simulink model "nn_fuel_control_4_15"  (R2021a)
settings: Solver=ode15s  StartTime=0.0  StopTime=T  MaxStep=.01  RelTol=1e-3
undefined symbols (not defined in the file): AF_sensor_tol, fault_time, fuel_inj_tol, kappa_tol, MAF_sensor_tol, pump_tol, tau_ww_tol
libraries: neural x66
(part 2 of 3)

== system nn_fuel_control_4_15/Air Fuel Control Model 1/Feed-Forward Neural Network/Layer 2/Delays 1 ==
  "p{2}" : Inport  PortDimensions=15
      mask Display: e = 0.06;c1 = [120 230 180]/255;c2 = ([120 230 180]+0)/(256+128);c3 = ([120 230 180]+128)/(256+128);patch([0 1 1 0],[0 0 1 1],c1);patch([0 1 1 1-e 1-e 0+e],[0 0 1 1-e 0+e 0+e],c2);patch([0 0 1 1-e 0+e 0+e],[0 1 1 1-e 1-e 0+e],c3);plot([0 1 1 0 0],[0 0 1 1 0]);
  mux : Mux  Inputs=1
      mask Display: e = 0.06;c1 = [120 150 230]/255;c2 = ([120 150 230]+0)/383;c3 = ([120 150 230]+128)/383;patch([0 1 1 0],[0 0 1 1],c1);patch([0 1 1 1-e 1-e 0+e],[0 0 1 1-e 0+e 0+e],c2);patch([0 0 1 1-e 0+e 0+e],[0 1 1 1-e 1-e 0+e],c3);plot([0 1 1 0 0],[0 0 1 1 0]);disp('Mux')
  "pd{2,1}" : Outport
      mask Display: e = 0.06;c1 = [120 230 180]/255;c2 = ([120 230 180]+0)/(256+128);c3 = ([120 230 180]+128)/(256+128);patch([0 1 1 0],[0 0 1 1],c1);patch([0 1 1 1-e 1-e 0+e],[0 0 1 1-e 0+e 0+e],c2);patch([0 0 1 1-e 0+e 0+e],[0 1 1 1-e 1-e 0+e],c3);plot([0 1 1 0 0],[0 0 1 1 0]);
  wires:
  "p{2}"/1 -> mux/1
  mux/1 -> "pd{2,1}"/1

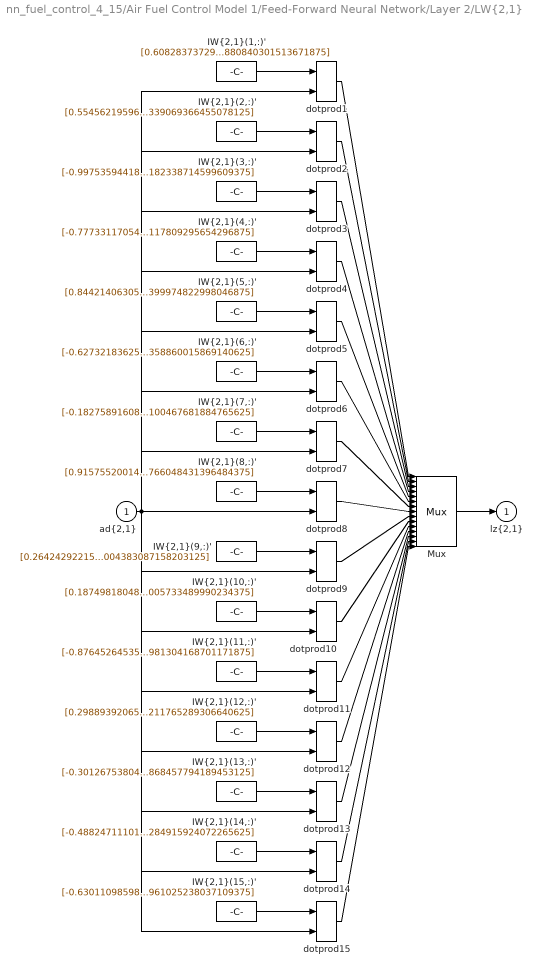
== system nn_fuel_control_4_15/Air Fuel Control Model 1/Feed-Forward Neural Network/Layer 2/LW{2,1} ==
  "ad{2,1}" : Inport  PortDimensions=15
      mask Display: e = 0.06;c1 = [120 230 180]/255;c2 = ([120 230 180]+0)/(256+128);c3 = ([120 230 180]+128)/(256+128);patch([0 1 1 0],[0 0 1 1],c1);patch([0 1 1 1-e 1-e 0+e],[0 0 1 1-e 0+e 0+e],c2);patch([0 0 1 1-e 0+e 0+e],[0 1 1 1-e 1-e 0+e],c3);plot([0 1 1 0 0],[0 0 1 1 0]);
  "IW{2,1}(1,:)'" : Constant  Value=[0.60828373729495710531267604892491362988948822021484375;0.1631652431061806074463760296566761098802089691162109375;-0.44374590709596450910368048425880260765552520751953125;0.345526680299295285703209401617641560733318328857421875;0.348097898689621876311406367676681838929653167724609375;0.8265636312091990678396768998936749994754791259765625;-0.01586618016159375976759093873624806292355060577392578125;0.6795632649425040749946447249385528266429901123046875;0.75459019889386735879810430560610257089138031005859375;-0.94837435293727867513524643072742037475109100341796875;-0.14339378395662694121170943617471493780612945556640625;0.1155478101778000254995504292310215532779693603515625;0.032676095155037145068011028570253984071314334869384765625;0.719801219521268631496013767900876700878143310546875;-0.5649534439609567026963077296386472880840301513671875]
      mask Display: e = 0.06;c1 = [120 150 230]/255;c2 = ([120 150 230]+0)/383;c3 = ([120 150 230]+128)/383;patch([0 1 1 0],[0 0 1 1],c1);patch([0 1 1 1-e 1-e 0+e],[0 0 1 1-e 0+e 0+e],c2);patch([0 0 1 1-e 0+e 0+e],[0 1 1 1-e 1-e 0+e],c3);plot([0 1 1 0 0],[0 0 1 1 0]);disp('weights');
  "IW{2,1}(10,:)'" : Constant  Value=[0.1874981804874335244992522575557813979685306549072265625;-0.387364613522674650081256686462438665330410003662109375;0.78290743200496437648183700730442069470882415771484375;0.86317824192602399246965205747983418405055999755859375;-0.59813734503873805525842044517048634588718414306640625;0.3906864891603387679452907832455821335315704345703125;-0.8173791825222698204100879593170247972011566162109375;0.9015721689759768064931222397717647254467010498046875;-0.146378292631031692305754177141352556645870208740234375;0.53947856391638715489733613139833323657512664794921875;-0.709668238586643074228277328074909746646881103515625;0.04455141979717640310365567302142153494060039520263671875;0.6061687426195963013242362649179995059967041015625;0.0751321602491212825469801828148774802684783935546875;0.478851095922558922524103763862513005733489990234375]
      mask Display: e = 0.06;c1 = [120 150 230]/255;c2 = ([120 150 230]+0)/383;c3 = ([120 150 230]+128)/383;patch([0 1 1 0],[0 0 1 1],c1);patch([0 1 1 1-e 1-e 0+e],[0 0 1 1-e 0+e 0+e],c2);patch([0 0 1 1-e 0+e 0+e],[0 1 1 1-e 1-e 0+e],c3);plot([0 1 1 0 0],[0 0 1 1 0]);disp('weights');
  "IW{2,1}(11,:)'" : Constant  Value=[-0.87645264535886735490777255108696408569812774658203125;-0.354803487782416215878811271977610886096954345703125;0.89745590027941080091267167517798952758312225341796875;0.12153107756977178655066751389313139952719211578369140625;0.0263130815585567445769044070402742363512516021728515625;-0.809370187848432731669845452415756881237030029296875;-0.50487186526927352314686459067161194980144500732421875;0.263576711957190124024918986833654344081878662109375;0.7429357474631868019088187793386168777942657470703125;0.12413592320170453719985204088516184128820896148681640625;0.12395570443307211971895043234326294623315334320068359375;-0.09320289501976443402586625097683281637728214263916015625;0.2053486431587812355292754773472552187740802764892578125;-0.14973778798840076120768571854569017887115478515625;-0.935185280441018118580132068018428981304168701171875]
      mask Display: e = 0.06;c1 = [120 150 230]/255;c2 = ([120 150 230]+0)/383;c3 = ([120 150 230]+128)/383;patch([0 1 1 0],[0 0 1 1],c1);patch([0 1 1 1-e 1-e 0+e],[0 0 1 1-e 0+e 0+e],c2);patch([0 0 1 1-e 0+e 0+e],[0 1 1 1-e 1-e 0+e],c3);plot([0 1 1 0 0],[0 0 1 1 0]);disp('weights');
  "IW{2,1}(12,:)'" : Constant  Value=[0.298893920656925160539429953132639639079570770263671875;-0.943158196479241706100538067403249442577362060546875;-0.72901934273769131156228695544996298849582672119140625;-0.4420743609879778102111913540284149348735809326171875;0.162898079805751105908484532847069203853607177734375;-0.03893962992941624179366044700145721435546875;-0.0249149427296144754251372432918287813663482666015625;0.7848685910094259643443592722178436815738677978515625;-0.7452172890261443694015497385407797992229461669921875;0.5937912927176427491104959699441678822040557861328125;-0.6901888632454264982385438997880555689334869384765625;0.297856720876973513068008969639777205884456634521484375;0.5644902002231066973081397009082138538360595703125;-0.1919252452819204535217068041674792766571044921875;0.955896418076493947779681548126973211765289306640625]
      mask Display: e = 0.06;c1 = [120 150 230]/255;c2 = ([120 150 230]+0)/383;c3 = ([120 150 230]+128)/383;patch([0 1 1 0],[0 0 1 1],c1);patch([0 1 1 1-e 1-e 0+e],[0 0 1 1-e 0+e 0+e],c2);patch([0 0 1 1-e 0+e 0+e],[0 1 1 1-e 1-e 0+e],c3);plot([0 1 1 0 0],[0 0 1 1 0]);disp('weights');
  "IW{2,1}(13,:)'" : Constant  Value=[-0.301267538043442584250186655481229536235332489013671875;0.2137960673758446950021294696853146888315677642822265625;-0.6099118162917822605351148013141937553882598876953125;-0.804913922659836078565831485320813953876495361328125;-0.77569083568485186486185511967050842940807342529296875;-0.1203229492733475236576623501605354249477386474609375;-0.4309096198696529267380128658260218799114227294921875;0.4020616862706465344245998494443483650684356689453125;0.8648307403643740176590881674201227724552154541015625;-0.7468845527558245489530008853762410581111907958984375;0.856263604397531796763587408349849283695220947265625;-0.9225328397592240659008666625595651566982269287109375;0.9259027011481022473304847153485752642154693603515625;0.567169309423982692663912530406378209590911865234375;-0.2729640593072322207746083222446031868457794189453125]
      mask Display: e = 0.06;c1 = [120 150 230]/255;c2 = ([120 150 230]+0)/383;c3 = ([120 150 230]+128)/383;patch([0 1 1 0],[0 0 1 1],c1);patch([0 1 1 1-e 1-e 0+e],[0 0 1 1-e 0+e 0+e],c2);patch([0 0 1 1-e 0+e 0+e],[0 1 1 1-e 1-e 0+e],c3);plot([0 1 1 0 0],[0 0 1 1 0]);disp('weights');
  "IW{2,1}(14,:)'" : Constant  Value=[-0.4882471110167276862057406106032431125640869140625;-0.153288731021647084418191298027522861957550048828125;0.42935429919651912911149338469840586185455322265625;-0.9702630312509814558552534435875713825225830078125;0.3583641699961483961800468023284338414669036865234375;-0.1353416572083896429745664136135019361972808837890625;0.4918952919432595383142370337736792862415313720703125;-0.57640236234023856098929172731004655361175537109375;-0.8508523606948406037275844937539659440517425537109375;-0.0224638760367827927666439791209995746612548828125;-0.095033702909726347485275255166925489902496337890625;0.8424006088431996719378958005108870565891265869140625;-0.6849380364954396060994668005150742828845977783203125;0.6228510334032935080728066168376244604587554931640625;-0.4631992710325454343234241605387069284915924072265625]
      mask Display: e = 0.06;c1 = [120 150 230]/255;c2 = ([120 150 230]+0)/383;c3 = ([120 150 230]+128)/383;patch([0 1 1 0],[0 0 1 1],c1);patch([0 1 1 1-e 1-e 0+e],[0 0 1 1-e 0+e 0+e],c2);patch([0 0 1 1-e 0+e 0+e],[0 1 1 1-e 1-e 0+e],c3);plot([0 1 1 0 0],[0 0 1 1 0]);disp('weights');
  "IW{2,1}(15,:)'" : Constant  Value=[-0.630110985981365612218496607965789735317230224609375;0.8242276349657886580502008655457757413387298583984375;-0.400759189777235125262677684077061712741851806640625;0.3277466841598546398728331041638739407062530517578125;0.8915540017782561665882212764699943363666534423828125;0.83874918710984758263293770141899585723876953125;0.45485624724982631761349693988449871540069580078125;0.4460472529162602395302883451222442090511322021484375;0.093826789799659859880875956150703132152557373046875;-0.9259823634579957829515706180245615541934967041015625;0.402471624402540584242160548456013202667236328125;-0.3445278733840286822243115238961763679981231689453125;-0.74855326961618029457667944370768964290618896484375;0.95153598362676117261571562266908586025238037109375;0.9375332121621331449290437376475892961025238037109375]
      mask Display: e = 0.06;c1 = [120 150 230]/255;c2 = ([120 150 230]+0)/383;c3 = ([120 150 230]+128)/383;patch([0 1 1 0],[0 0 1 1],c1);patch([0 1 1 1-e 1-e 0+e],[0 0 1 1-e 0+e 0+e],c2);patch([0 0 1 1-e 0+e 0+e],[0 1 1 1-e 1-e 0+e],c3);plot([0 1 1 0 0],[0 0 1 1 0]);disp('weights');
  "IW{2,1}(2,:)'" : Constant  Value=[0.554562195967324811363141634501516819000244140625;0.1497692577584186779393604638244141824543476104736328125;0.56295505738794149319659254615544341504573822021484375;-0.79339302952488333087188721037819050252437591552734375;-0.5227228745047407532098304727696813642978668212890625;-0.3416227507267695084891556689399294555187225341796875;-0.077931032288060197998902367544360458850860595703125;0.791132526371828515010520277428440749645233154296875;-0.58148454694741247283928942124475724995136260986328125;0.141240162213906061960955184986232779920101165771484375;-0.47295622510494939039205064545967616140842437744140625;-0.88474738325846635778049176224158145487308502197265625;-0.2412424077947986911230060513844364322721958160400390625;0.026695649520263042830947597394697368144989013671875;-0.168815586171824794092799493228085339069366455078125]
      mask Display: e = 0.06;c1 = [120 150 230]/255;c2 = ([120 150 230]+0)/383;c3 = ([120 150 230]+128)/383;patch([0 1 1 0],[0 0 1 1],c1);patch([0 1 1 1-e 1-e 0+e],[0 0 1 1-e 0+e 0+e],c2);patch([0 0 1 1-e 0+e 0+e],[0 1 1 1-e 1-e 0+e],c3);plot([0 1 1 0 0],[0 0 1 1 0]);disp('weights');
  "IW{2,1}(3,:)'" : Constant  Value=[-0.997535944186512590903248565155081450939178466796875;0.9844775557991563008641833221190609037876129150390625;0.13365057898997889651582227088510990142822265625;0.598462918022267142958980912226252257823944091796875;-0.6928984585121236161597835234715603291988372802734375;0.47725275298145408697791935992427170276641845703125;0.31490478145201183934887012583203613758087158203125;-0.596507724440733522186519621754996478557586669921875;0.00503819451104714488565150531940162181854248046875;-0.1558413435872125774039886891841888427734375;0.069703488503479515969729618518613278865814208984375;0.252706700102361292437080919626168906688690185546875;0.6096076508018011264056212894502095878124237060546875;-0.6419028490453777546775882001384161412715911865234375;0.809099317995565225913878748542629182338714599609375]
      mask Display: e = 0.06;c1 = [120 150 230]/255;c2 = ([120 150 230]+0)/383;c3 = ([120 150 230]+128)/383;patch([0 1 1 0],[0 0 1 1],c1);patch([0 1 1 1-e 1-e 0+e],[0 0 1 1-e 0+e 0+e],c2);patch([0 0 1 1-e 0+e 0+e],[0 1 1 1-e 1-e 0+e],c3);plot([0 1 1 0 0],[0 0 1 1 0]);disp('weights');
  "IW{2,1}(4,:)'" : Constant  Value=[-0.7773311705499761359305921359919011592864990234375;-0.1463969306597807662484456159290857613086700439453125;-0.52098250625950992542811945895664393901824951171875;0.1340370775561925409391506036627106368541717529296875;0.286894704491670982093864950002171099185943603515625;-0.2232587156037413311793216053047217428684234619140625;0.30007640022437698235080461017787456512451171875;-0.587710092220042223942755299503915011882781982421875;0.3578658787775890193216810075682587921619415283203125;-0.2262986592885329883984013576991856098175048828125;-0.658201336972639605704671339481137692928314208984375;-0.2545120319323490587493097336846403777599334716796875;-0.2189509488661911529305825752089731395244598388671875;-0.1927993718650127252800530186505056917667388916015625;0.31411982797593207550335137057118117809295654296875]
      mask Display: e = 0.06;c1 = [120 150 230]/255;c2 = ([120 150 230]+0)/383;c3 = ([120 150 230]+128)/383;patch([0 1 1 0],[0 0 1 1],c1);patch([0 1 1 1-e 1-e 0+e],[0 0 1 1-e 0+e 0+e],c2);patch([0 0 1 1-e 0+e 0+e],[0 1 1 1-e 1-e 0+e],c3);plot([0 1 1 0 0],[0 0 1 1 0]);disp('weights');
  "IW{2,1}(5,:)'" : Constant  Value=[0.8442140630590719840853353161946870386600494384765625;-0.338275289571432880020296352086006663739681243896484375;0.78093285572494230972750983710284344851970672607421875;0.5354024127678302935606780010857619345188140869140625;-0.08976512545403049492254154984038905240595340728759765625;0.0061947204318573145798154655494727194309234619140625;-0.66291433016892231666616908114519901573657989501953125;-0.0206699629090130176933826078311540186405181884765625;-0.59971454427786785590370755016920156776905059814453125;0.10166800703172866604528934431073139421641826629638671875;-0.7738583581044451431552033682237379252910614013671875;0.54327144951764783087355681345798075199127197265625;-0.7895437576381787447843407790060155093669891357421875;-0.264681039126205330802577009308151900768280029296875;-0.531626874309292229980883348616771399974822998046875]
      mask Display: e = 0.06;c1 = [120 150 230]/255;c2 = ([120 150 230]+0)/383;c3 = ([120 150 230]+128)/383;patch([0 1 1 0],[0 0 1 1],c1);patch([0 1 1 1-e 1-e 0+e],[0 0 1 1-e 0+e 0+e],c2);patch([0 0 1 1-e 0+e 0+e],[0 1 1 1-e 1-e 0+e],c3);plot([0 1 1 0 0],[0 0 1 1 0]);disp('weights');
  "IW{2,1}(6,:)'" : Constant  Value=[-0.6273218362596340025305607923655770719051361083984375;0.656185430676088810031387765775434672832489013671875;0.811438500319960898110593916499055922031402587890625;0.6995755518931172645125116105191409587860107421875;-0.1562054093044125957501222501377924345433712005615234375;-0.0322626762571427416759206607821397483348846435546875;-0.01132390864387658978296169465238563134334981441497802734375;-0.4057941893418341994248521586996503174304962158203125;0.70209822919968012389091427394305355846881866455078125;-0.6537984598108443901054442903841845691204071044921875;-0.53447697884651301780678522845846600830554962158203125;0.9945723398383783386833556505735032260417938232421875;-0.168349065817595733296485605023917742073535919189453125;-0.164941923712752736008724241401068866252899169921875;0.071348316420243751423413414158858358860015869140625]
      mask Display: e = 0.06;c1 = [120 150 230]/255;c2 = ([120 150 230]+0)/383;c3 = ([120 150 230]+128)/383;patch([0 1 1 0],[0 0 1 1],c1);patch([0 1 1 1-e 1-e 0+e],[0 0 1 1-e 0+e 0+e],c2);patch([0 0 1 1-e 0+e 0+e],[0 1 1 1-e 1-e 0+e],c3);plot([0 1 1 0 0],[0 0 1 1 0]);disp('weights');
  "IW{2,1}(7,:)'" : Constant  Value=[-0.1827589160867006956578961762716062366962432861328125;0.264553209549575729653270173002965748310089111328125;-0.602076083278996865288945627980865538120269775390625;-0.8668388126716621844281007724930532276630401611328125;-0.631703471288605822309136783587746322154998779296875;0.738811602164048064622647871146909892559051513671875;-0.29851980211238693385666920221410691738128662109375;-0.9066514471495474847273499108268879354000091552734375;0.7667373784025228733440826545120216906070709228515625;-0.8003713287638996032313798423274420201778411865234375;0.572112014899465837203251794562675058841705322265625;0.0556726723526870248548448216752149164676666259765625;0.1886458668441315378316858186735771596431732177734375;-0.43769519159423087018012665794230997562408447265625;0.2958829770965698546802968849078752100467681884765625]
      mask Display: e = 0.06;c1 = [120 150 230]/255;c2 = ([120 150 230]+0)/383;c3 = ([120 150 230]+128)/383;patch([0 1 1 0],[0 0 1 1],c1);patch([0 1 1 1-e 1-e 0+e],[0 0 1 1-e 0+e 0+e],c2);patch([0 0 1 1-e 0+e 0+e],[0 1 1 1-e 1-e 0+e],c3);plot([0 1 1 0 0],[0 0 1 1 0]);disp('weights');
  "IW{2,1}(8,:)'" : Constant  Value=[0.9157552001415154574459620562265627086162567138671875;0.1691210332467132648748275869365897960960865020751953125;-0.410972009283113226540962159560876898467540740966796875;-0.79231054870772366083286897264770232141017913818359375;-0.6664760715628090803619443249772302806377410888671875;0.4958051958545179882520415048929862678050994873046875;0.8372202716459440363649946448276750743389129638671875;-0.6574527075494429606550284006516449153423309326171875;0.20364663569650731655968911582021974027156829833984375;0.477164411668982768599533983433502726256847381591796875;0.2366940977861309580720927669972297735512256622314453125;-0.137137595850200855185363479904481209814548492431640625;-0.0219191390002913925882932488775622914545238018035888671875;-0.414790307653978285173934636986814439296722412109375;0.2688907245261178413642255691229365766048431396484375]
      mask Display: e = 0.06;c1 = [120 150 230]/255;c2 = ([120 150 230]+0)/383;c3 = ([120 150 230]+128)/383;patch([0 1 1 0],[0 0 1 1],c1);patch([0 1 1 1-e 1-e 0+e],[0 0 1 1-e 0+e 0+e],c2);patch([0 0 1 1-e 0+e 0+e],[0 1 1 1-e 1-e 0+e],c3);plot([0 1 1 0 0],[0 0 1 1 0]);disp('weights');
  "IW{2,1}(9,:)'" : Constant  Value=[0.264242922159276749649592375135398469865322113037109375;0.0281964884631230143507973906480401637963950634002685546875;0.437970352052139799692298538502654992043972015380859375;0.85719086127498778093780629205866716802120208740234375;0.6149400332096350840771492585190571844577789306640625;-0.1298886743902054607957552434527315199375152587890625;-0.116547252626436392830555632826872169971466064453125;-0.99659741931905632128518846002407371997833251953125;-0.19318002865432382098020980265573598444461822509765625;-0.8425582572983163487378988065756857395172119140625;0.1149262515205252410677161378771415911614894866943359375;0.73176535852285640171288605415611527860164642333984375;-0.2544570268941874768842126286472193896770477294921875;0.66147788735934387460702055250294506549835205078125;-0.688203072177270502862711509806104004383087158203125]
      mask Display: e = 0.06;c1 = [120 150 230]/255;c2 = ([120 150 230]+0)/383;c3 = ([120 150 230]+128)/383;patch([0 1 1 0],[0 0 1 1],c1);patch([0 1 1 1-e 1-e 0+e],[0 0 1 1-e 0+e 0+e],c2);patch([0 0 1 1-e 0+e 0+e],[0 1 1 1-e 1-e 0+e],c3);plot([0 1 1 0 0],[0 0 1 1 0]);disp('weights');
  Mux : Mux  Inputs=15
      mask Display: e = 0.06;c1 = [120 150 230]/255;c2 = ([120 150 230]+0)/383;c3 = ([120 150 230]+128)/383;patch([0 1 1 0],[0 0 1 1],c1);patch([0 1 1 1-e 1-e 0+e],[0 0 1 1-e 0+e 0+e],c2);patch([0 0 1 1-e 0+e 0+e],[0 1 1 1-e 1-e 0+e],c3);plot([0 1 1 0 0],[0 0 1 1 0]);disp('Mux');
  dotprod{1..15} (15 alike) : neural/Weight Functions/dotprod
  "lz{2,1}" : Outport
      mask Display: e = 0.06;c1 = [120 230 180]/255;c2 = ([120 230 180]+0)/(256+128);c3 = ([120 230 180]+128)/(256+128);patch([0 1 1 0],[0 0 1 1],c1);patch([0 1 1 1-e 1-e 0+e],[0 0 1 1-e 0+e 0+e],c2);patch([0 0 1 1-e 0+e 0+e],[0 1 1 1-e 1-e 0+e],c3);plot([0 1 1 0 0],[0 0 1 1 0]);
  wires:
  "IW{2,1}(1,:)'"/1 -> dotprod1/1
  "ad{2,1}"/1 -> dotprod1/2, dotprod2/2, dotprod3/2, dotprod4/2, dotprod5/2, dotprod6/2, dotprod7/2, dotprod8/2, dotprod9/2, dotprod10/2, dotprod11/2, dotprod12/2, dotprod13/2, dotprod14/2, dotprod15/2
  dotprod1/1 -> Mux/1
  "IW{2,1}(2,:)'"/1 -> dotprod2/1
  dotprod2/1 -> Mux/2
  "IW{2,1}(3,:)'"/1 -> dotprod3/1
  dotprod3/1 -> Mux/3
  "IW{2,1}(4,:)'"/1 -> dotprod4/1
  dotprod4/1 -> Mux/4
  "IW{2,1}(5,:)'"/1 -> dotprod5/1
  dotprod5/1 -> Mux/5
  "IW{2,1}(6,:)'"/1 -> dotprod6/1
  dotprod6/1 -> Mux/6
  "IW{2,1}(7,:)'"/1 -> dotprod7/1
  dotprod7/1 -> Mux/7
  "IW{2,1}(8,:)'"/1 -> dotprod8/1
  dotprod8/1 -> Mux/8
  "IW{2,1}(9,:)'"/1 -> dotprod9/1
  dotprod9/1 -> Mux/9
  "IW{2,1}(10,:)'"/1 -> dotprod10/1
  dotprod10/1 -> Mux/10
  "IW{2,1}(11,:)'"/1 -> dotprod11/1
  dotprod11/1 -> Mux/11
  "IW{2,1}(12,:)'"/1 -> dotprod12/1
  dotprod12/1 -> Mux/12
  "IW{2,1}(13,:)'"/1 -> dotprod13/1
  dotprod13/1 -> Mux/13
  "IW{2,1}(14,:)'"/1 -> dotprod14/1
  dotprod14/1 -> Mux/14
  "IW{2,1}(15,:)'"/1 -> dotprod15/1
  dotprod15/1 -> Mux/15
  Mux/1 -> "lz{2,1}"/1

== system nn_fuel_control_4_15/Air Fuel Control Model 1/Feed-Forward Neural Network/Layer 3/Delays 1 ==
  "p{3}" : Inport  PortDimensions=15
      mask Display: e = 0.06;c1 = [120 230 180]/255;c2 = ([120 230 180]+0)/(256+128);c3 = ([120 230 180]+128)/(256+128);patch([0 1 1 0],[0 0 1 1],c1);patch([0 1 1 1-e 1-e 0+e],[0 0 1 1-e 0+e 0+e],c2);patch([0 0 1 1-e 0+e 0+e],[0 1 1 1-e 1-e 0+e],c3);plot([0 1 1 0 0],[0 0 1 1 0]);
  mux : Mux  Inputs=1
      mask Display: e = 0.06;c1 = [120 150 230]/255;c2 = ([120 150 230]+0)/383;c3 = ([120 150 230]+128)/383;patch([0 1 1 0],[0 0 1 1],c1);patch([0 1 1 1-e 1-e 0+e],[0 0 1 1-e 0+e 0+e],c2);patch([0 0 1 1-e 0+e 0+e],[0 1 1 1-e 1-e 0+e],c3);plot([0 1 1 0 0],[0 0 1 1 0]);disp('Mux')
  "pd{3,2}" : Outport
      mask Display: e = 0.06;c1 = [120 230 180]/255;c2 = ([120 230 180]+0)/(256+128);c3 = ([120 230 180]+128)/(256+128);patch([0 1 1 0],[0 0 1 1],c1);patch([0 1 1 1-e 1-e 0+e],[0 0 1 1-e 0+e 0+e],c2);patch([0 0 1 1-e 0+e 0+e],[0 1 1 1-e 1-e 0+e],c3);plot([0 1 1 0 0],[0 0 1 1 0]);
  wires:
  "p{3}"/1 -> mux/1
  mux/1 -> "pd{3,2}"/1

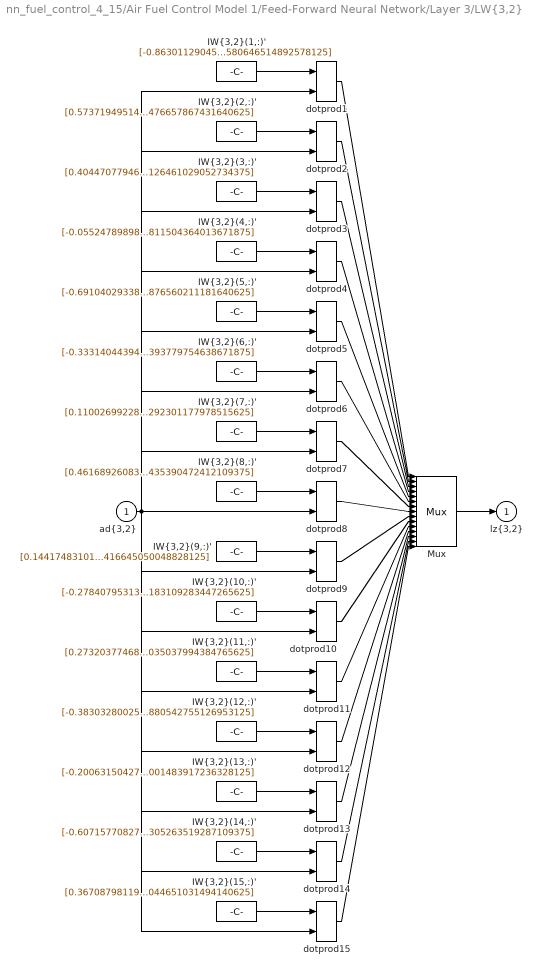
== system nn_fuel_control_4_15/Air Fuel Control Model 1/Feed-Forward Neural Network/Layer 3/LW{3,2} ==
  "ad{3,2}" : Inport  PortDimensions=15
      mask Display: e = 0.06;c1 = [120 230 180]/255;c2 = ([120 230 180]+0)/(256+128);c3 = ([120 230 180]+128)/(256+128);patch([0 1 1 0],[0 0 1 1],c1);patch([0 1 1 1-e 1-e 0+e],[0 0 1 1-e 0+e 0+e],c2);patch([0 0 1 1-e 0+e 0+e],[0 1 1 1-e 1-e 0+e],c3);plot([0 1 1 0 0],[0 0 1 1 0]);
  "IW{3,2}(1,:)'" : Constant  Value=[-0.86301129045804658712626178385107778012752532958984375;0.6118016357822815276534811346209608018398284912109375;-0.448770468717050174944915852393023669719696044921875;0.039417878855195542797673624590970575809478759765625;-0.272599409373730505734556572861038148403167724609375;-0.0132278525814354432077468715078794048167765140533447265625;0.27510893551842041659938331576995551586151123046875;-0.162565749757493327454227483030990697443485260009765625;0.86779513409330311102252153432345949113368988037109375;0.20707874169687523480121171814971603453159332275390625;0.66311428716604814415092050694511272013187408447265625;-0.7740931133928767859941899587283842265605926513671875;-0.86487600584277257720344778135768137872219085693359375;0.9661205861212127654624737260746769607067108154296875;0.021058795368890770305370097048580646514892578125]
      mask Display: e = 0.06;c1 = [120 150 230]/255;c2 = ([120 150 230]+0)/383;c3 = ([120 150 230]+128)/383;patch([0 1 1 0],[0 0 1 1],c1);patch([0 1 1 1-e 1-e 0+e],[0 0 1 1-e 0+e 0+e],c2);patch([0 0 1 1-e 0+e 0+e],[0 1 1 1-e 1-e 0+e],c3);plot([0 1 1 0 0],[0 0 1 1 0]);disp('weights');
  "IW{3,2}(10,:)'" : Constant  Value=[-0.2784079531374601401694235391914844512939453125;0.608168294583068647085610791691578924655914306640625;0.4652128874334693353631564605166204273700714111328125;0.2117353163302924112798564237891696393489837646484375;-0.3877434427272914430062655810615979135036468505859375;0.2567645318176783320041067781858146190643310546875;-0.9876800453373617560970387785346247255802154541015625;0.5191759503268860154179265009588561952114105224609375;0.17881360392462664066215438651852309703826904296875;-0.762561135099049547392269232659600675106048583984375;-0.3519010091170191589782234586891718208789825439453125;0.7049522434356412237121958241914398968219757080078125;-0.1176158877623338927520535435178317129611968994140625;0.299986772273917789988217919017188251018524169921875;-0.1147249348728200946112565361545421183109283447265625]
      mask Display: e = 0.06;c1 = [120 150 230]/255;c2 = ([120 150 230]+0)/383;c3 = ([120 150 230]+128)/383;patch([0 1 1 0],[0 0 1 1],c1);patch([0 1 1 1-e 1-e 0+e],[0 0 1 1-e 0+e 0+e],c2);patch([0 0 1 1-e 0+e 0+e],[0 1 1 1-e 1-e 0+e],c3);plot([0 1 1 0 0],[0 0 1 1 0]);disp('weights');
  "IW{3,2}(11,:)'" : Constant  Value=[0.273203774685698619340001869204570539295673370361328125;-0.7906595053305698339585205758339725434780120849609375;0.583849070000980407968427243758924305438995361328125;0.9383988246397245713836809954955242574214935302734375;-0.66072231702565542565963596643996424973011016845703125;-0.891472443481964749167900663451291620731353759765625;0.7874416108864068508665923218359239399433135986328125;0.5926967993300336079443013659329153597354888916015625;1.0150000646592898245756941832951270043849945068359375;-0.49763449710267126935292480993666686117649078369140625;0.8673541032724652044549884521984495222568511962890625;-0.8384421201588592165165891856304369866847991943359375;-0.83482001699344998701945996799622662365436553955078125;0.690854562472308142417887211195193231105804443359375;-0.6268860403933749214644421954290010035037994384765625]
      mask Display: e = 0.06;c1 = [120 150 230]/255;c2 = ([120 150 230]+0)/383;c3 = ([120 150 230]+128)/383;patch([0 1 1 0],[0 0 1 1],c1);patch([0 1 1 1-e 1-e 0+e],[0 0 1 1-e 0+e 0+e],c2);patch([0 0 1 1-e 0+e 0+e],[0 1 1 1-e 1-e 0+e],c3);plot([0 1 1 0 0],[0 0 1 1 0]);disp('weights');
  "IW{3,2}(12,:)'" : Constant  Value=[-0.3830328002595309033750936578144319355487823486328125;0.5655287131020296786942935796105302870273590087890625;-0.56563755415870264897648667101748287677764892578125;-0.753895819854298654405511115328408777713775634765625;0.107689861230984007534061674959957599639892578125;-0.8865608902806403346374963803100399672985076904296875;-0.5902057650183234471796822617761790752410888671875;-0.1535974223764247081902567515498958528041839599609375;-0.867548499667184724870594436652027070522308349609375;0.6646644756044224333635384027729742228984832763671875;0.9682276139976793150054845682461746037006378173828125;-0.5334045222875605229972961751627735793590545654296875;0.4884919333138866281984746819944120943546295166015625;0.029331742387500359114937964477576315402984619140625;-0.977416297114818366509325642255134880542755126953125]
      mask Display: e = 0.06;c1 = [120 150 230]/255;c2 = ([120 150 230]+0)/383;c3 = ([120 150 230]+128)/383;patch([0 1 1 0],[0 0 1 1],c1);patch([0 1 1 1-e 1-e 0+e],[0 0 1 1-e 0+e 0+e],c2);patch([0 0 1 1-e 0+e 0+e],[0 1 1 1-e 1-e 0+e],c3);plot([0 1 1 0 0],[0 0 1 1 0]);disp('weights');
  "IW{3,2}(13,:)'" : Constant  Value=[-0.20063150427935616537666874137357808649539947509765625;-0.769446195419788647740233500371687114238739013671875;0.485845181970760986445156959234736859798431396484375;-0.084858866708749314256010620738379657268524169921875;0.61400264595550535506873757185530848801136016845703125;0.5329320363735552401607264982885681092739105224609375;0.8255560603635421212942446800298057496547698974609375;-0.7469931562344085396176751601160503923892974853515625;0.76459182355636468031434560543857514858245849609375;-0.796321636595974435834932592115364968776702880859375;0.59767623864360641672277552061132155358791351318359375;-0.72224027678053259737822600072831846773624420166015625;0.75478704374997318549134206477901898324489593505859375;-0.30987484137478649159902488463558256626129150390625;-0.59844341974986026144733841647394001483917236328125]
      mask Display: e = 0.06;c1 = [120 150 230]/255;c2 = ([120 150 230]+0)/383;c3 = ([120 150 230]+128)/383;patch([0 1 1 0],[0 0 1 1],c1);patch([0 1 1 1-e 1-e 0+e],[0 0 1 1-e 0+e 0+e],c2);patch([0 0 1 1-e 0+e 0+e],[0 1 1 1-e 1-e 0+e],c3);plot([0 1 1 0 0],[0 0 1 1 0]);disp('weights');
  "IW{3,2}(14,:)'" : Constant  Value=[-0.6071577082703163430466020145104266703128814697265625;-0.977261163813881950090944883413612842559814453125;0.26082563918290357918294830597005784511566162109375;-0.5621206550281094838084072762285359203815460205078125;0.781323428675917863728273005108349025249481201171875;-0.9882329094186397266952326390310190618038177490234375;0.334472346623993388448070618323981761932373046875;-0.464401218551299788117603384307585656642913818359375;-0.643436170363963721996469757868908345699310302734375;0.5020371182082949967906415622564963996410369873046875;0.882280327269156838809749388019554316997528076171875;0.50220598748147526890761582762934267520904541015625;-0.01116367837432985510304206400178372859954833984375;0.89157101398662330637989725801162421703338623046875;0.58068507151349191275357952690683305263519287109375]
      mask Display: e = 0.06;c1 = [120 150 230]/255;c2 = ([120 150 230]+0)/383;c3 = ([120 150 230]+128)/383;patch([0 1 1 0],[0 0 1 1],c1);patch([0 1 1 1-e 1-e 0+e],[0 0 1 1-e 0+e 0+e],c2);patch([0 0 1 1-e 0+e 0+e],[0 1 1 1-e 1-e 0+e],c3);plot([0 1 1 0 0],[0 0 1 1 0]);disp('weights');
  "IW{3,2}(15,:)'" : Constant  Value=[0.367087981192719237100163809373043477535247802734375;-0.8840783120306510145525180632830597460269927978515625;-0.0580263017873499098442380272899754345417022705078125;0.971391528445162411031787996762432157993316650390625;0.654235661651310973496720180264674127101898193359375;0.5037187028825067525161784942611120641231536865234375;0.381673791584718369307438479154370725154876708984375;-0.52767635355878506064897237592958845198154449462890625;-0.289020960268621063260496839575353078544139862060546875;0.97031960554220020309657002144376747310161590576171875;-0.324301361004415367172981632393202744424343109130859375;-0.32842760696003114873064987477846443653106689453125;-0.90978766614605632856438433009316213428974151611328125;-0.244891135957543415457848823280073702335357666015625;0.0193583719873873238981332178809680044651031494140625]
      mask Display: e = 0.06;c1 = [120 150 230]/255;c2 = ([120 150 230]+0)/383;c3 = ([120 150 230]+128)/383;patch([0 1 1 0],[0 0 1 1],c1);patch([0 1 1 1-e 1-e 0+e],[0 0 1 1-e 0+e 0+e],c2);patch([0 0 1 1-e 0+e 0+e],[0 1 1 1-e 1-e 0+e],c3);plot([0 1 1 0 0],[0 0 1 1 0]);disp('weights');
  "IW{3,2}(2,:)'" : Constant  Value=[0.5737194951424340327861273181042633950710296630859375;-0.55584779618165924830464064143598079681396484375;-0.34954293145081738458657127921469509601593017578125;0.93717221057489208391189094982109963893890380859375;-0.94370267223165893444303264914196915924549102783203125;-0.535948676324559780681511256261728703975677490234375;-0.8093108252469212171575918546295724809169769287109375;0.83799835575733905290718439573538489639759063720703125;0.95074227019016432915776704248855821788311004638671875;0.10332739464158118003478392665783758275210857391357421875;0.7522640376001799022986915588262490928173065185546875;-0.699454141685345032186660318984650075435638427734375;0.2297571557743861292433251719558029435575008392333984375;-0.101376760179355596136474559898488223552703857421875;0.7655714832576736572633535615750588476657867431640625]
      mask Display: e = 0.06;c1 = [120 150 230]/255;c2 = ([120 150 230]+0)/383;c3 = ([120 150 230]+128)/383;patch([0 1 1 0],[0 0 1 1],c1);patch([0 1 1 1-e 1-e 0+e],[0 0 1 1-e 0+e 0+e],c2);patch([0 0 1 1-e 0+e 0+e],[0 1 1 1-e 1-e 0+e],c3);plot([0 1 1 0 0],[0 0 1 1 0]);disp('weights');
  "IW{3,2}(3,:)'" : Constant  Value=[0.404470779466199470419951467192731797695159912109375;0.60621496767803717542477670576772652566432952880859375;-0.0643392890122302940625331757473759353160858154296875;-0.1058288585889186617094992470811121165752410888671875;-0.65251687480068454316750603538821451365947723388671875;0.353378008209826621754956477161613292992115020751953125;0.0907164068557657632396740154945291578769683837890625;0.763843253698396562612060733954422175884246826171875;0.002443811284803519036368246730717146419920027256011962890625;0.70826898939199700588886798868770711123943328857421875;-0.00833867952434022043084471675911117927171289920806884765625;-0.58566340539244043927880056799040175974369049072265625;-0.98525597816140564333409201935864984989166259765625;0.7409087155778861788490985418320633471012115478515625;0.63190923572642443417635149671696126461029052734375]
      mask Display: e = 0.06;c1 = [120 150 230]/255;c2 = ([120 150 230]+0)/383;c3 = ([120 150 230]+128)/383;patch([0 1 1 0],[0 0 1 1],c1);patch([0 1 1 1-e 1-e 0+e],[0 0 1 1-e 0+e 0+e],c2);patch([0 0 1 1-e 0+e 0+e],[0 1 1 1-e 1-e 0+e],c3);plot([0 1 1 0 0],[0 0 1 1 0]);disp('weights');
  "IW{3,2}(4,:)'" : Constant  Value=[-0.05524789898072628158143260179713252000510692596435546875;-0.715980063590353932312382312375120818614959716796875;-0.24827863546763762059299551765434443950653076171875;-0.20919043727689601297470289864577353000640869140625;0.1430091727949580338030699522278155200183391571044921875;-0.60906711235546762139847487560473382472991943359375;-0.5117982914890959467157927065272815525531768798828125;0.75189667267167392683546722764731384813785552978515625;-0.799839899652887265091294466401450335979461669921875;0.953100423674601682222373710828833281993865966796875;0.0285665166643942029789382530680086347274482250213623046875;-0.450008619295558853767857954153441824018955230712890625;0.409533035675645196160843397592543624341487884521484375;0.4548305549922970758558449233532883226871490478515625;0.8436301244412163224950518269906751811504364013671875]
      mask Display: e = 0.06;c1 = [120 150 230]/255;c2 = ([120 150 230]+0)/383;c3 = ([120 150 230]+128)/383;patch([0 1 1 0],[0 0 1 1],c1);patch([0 1 1 1-e 1-e 0+e],[0 0 1 1-e 0+e 0+e],c2);patch([0 0 1 1-e 0+e 0+e],[0 1 1 1-e 1-e 0+e],c3);plot([0 1 1 0 0],[0 0 1 1 0]);disp('weights');
  "IW{3,2}(5,:)'" : Constant  Value=[-0.69104029338774619617424832540564239025115966796875;0.0040236846517431867908953790902160108089447021484375;0.8558400671177601726213879373972304165363311767578125;-0.895017775624558087343984880135394632816314697265625;-0.185095085071437015500350753427483141422271728515625;-0.4552171665127373589854187230230309069156646728515625;0.8776929106441315742159758883644826710224151611328125;0.130149489879824553639764417312107980251312255859375;-0.7703281021261820793455399325466714799404144287109375;-0.7694009645457742241347887102165259420871734619140625;0.6709251268978853044444576880778186023235321044921875;-0.561840735728180273866882998845539987087249755859375;-0.9573670871313069152819252849440090358257293701171875;0.65230071515839771478795228176750242710113525390625;0.69315907051306968611470438190735876560211181640625]
      mask Display: e = 0.06;c1 = [120 150 230]/255;c2 = ([120 150 230]+0)/383;c3 = ([120 150 230]+128)/383;patch([0 1 1 0],[0 0 1 1],c1);patch([0 1 1 1-e 1-e 0+e],[0 0 1 1-e 0+e 0+e],c2);patch([0 0 1 1-e 0+e 0+e],[0 1 1 1-e 1-e 0+e],c3);plot([0 1 1 0 0],[0 0 1 1 0]);disp('weights');
  "IW{3,2}(6,:)'" : Constant  Value=[-0.333140443941780828307486217454425059258937835693359375;-0.950103966495819296511626816936768591403961181640625;0.0581858891863988869630475164740346372127532958984375;-0.0021199494007231312053818328422494232654571533203125;0.425920052962606876523210530649521388113498687744140625;0.75380614628520259401511793839745223522186279296875;0.7716234645293440497226811203290708363056182861328125;0.99171021624842536912325385856092907488346099853515625;0.6294417293842882177301589763374067842960357666015625;0.7284246073046336533707290072925388813018798828125;0.95548261353571584120203397105797193944454193115234375;-0.9342151842929922178626611639629118144512176513671875;0.397697174578897805208299587320652790367603302001953125;0.5833037213148604127610497016576118767261505126953125;0.9831521234001427966830988225410692393779754638671875]
      mask Display: e = 0.06;c1 = [120 150 230]/255;c2 = ([120 150 230]+0)/383;c3 = ([120 150 230]+128)/383;patch([0 1 1 0],[0 0 1 1],c1);patch([0 1 1 1-e 1-e 0+e],[0 0 1 1-e 0+e 0+e],c2);patch([0 0 1 1-e 0+e 0+e],[0 1 1 1-e 1-e 0+e],c3);plot([0 1 1 0 0],[0 0 1 1 0]);disp('weights');
  "IW{3,2}(7,:)'" : Constant  Value=[0.110026992289163738636403877535485662519931793212890625;0.67373417683566449998266989496187306940555572509765625;-0.301845231266341773590511365910060703754425048828125;0.8019764531883470937145830248482525348663330078125;-0.11190227854424390774301656392708537168800830841064453125;0.67494032645118873237066736692213453352451324462890625;-0.5099673615384270330963545347913168370723724365234375;0.31292059457961551860449844753020443022251129150390625;-0.63635218605273247138853776050382293760776519775390625;0.96970856224714185866986326800542883574962615966796875;-0.359527703800834486091986264000297524034976959228515625;-0.41258192310656038870320116984657943248748779296875;0.484531410279573915289574870257638394832611083984375;-0.8836241928396517675281529591302387416362762451171875;-0.325175429526366688293137485743500292301177978515625]
      mask Display: e = 0.06;c1 = [120 150 230]/255;c2 = ([120 150 230]+0)/383;c3 = ([120 150 230]+128)/383;patch([0 1 1 0],[0 0 1 1],c1);patch([0 1 1 1-e 1-e 0+e],[0 0 1 1-e 0+e 0+e],c2);patch([0 0 1 1-e 0+e 0+e],[0 1 1 1-e 1-e 0+e],c3);plot([0 1 1 0 0],[0 0 1 1 0]);disp('weights');
  "IW{3,2}(8,:)'" : Constant  Value=[0.461689260835830783680222566545126028358936309814453125;-0.332442455427390537447962515216204337775707244873046875;0.45646483804751625257267733104526996612548828125;-0.2215993190882838970168222658685408532619476318359375;0.6560662726001549316379168885760009288787841796875;-0.92587183455379484797731493017636239528656005859375;-0.4386334251282750784639574703760445117950439453125;0.47009152133705589537981950343237258493900299072265625;0.308086259769605741443143642754876054823398590087890625;-0.0254944316844919159625870719310114509426057338714599609375;-0.6702147703875673823148417795891873538494110107421875;0.1605491516177627586703380302424193359911441802978515625;0.492253112905028211709890229030861519277095794677734375;-0.584491661139576734740330721251666545867919921875;0.58570920517953251049902974045835435390472412109375]
      mask Display: e = 0.06;c1 = [120 150 230]/255;c2 = ([120 150 230]+0)/383;c3 = ([120 150 230]+128)/383;patch([0 1 1 0],[0 0 1 1],c1);patch([0 1 1 1-e 1-e 0+e],[0 0 1 1-e 0+e 0+e],c2);patch([0 0 1 1-e 0+e 0+e],[0 1 1 1-e 1-e 0+e],c3);plot([0 1 1 0 0],[0 0 1 1 0]);disp('weights');
  "IW{3,2}(9,:)'" : Constant  Value=[0.144174831017278293199268546231905929744243621826171875;-0.07368648711068793988321345977965393103659152984619140625;0.5309182993399785832622228554100729525089263916015625;0.5905316342593065481736402944079600274562835693359375;-0.68450170306392810193329978574183769524097442626953125;0.62331332002594308505649678409099578857421875;0.9246864819524898138070057029835879802703857421875;0.33003678949862880198651282626087777316570281982421875;-0.058070114265279131060548678533450583927333354949951171875;0.292271144357206635877588496441603638231754302978515625;0.2078383392305152288503933277752366848289966583251953125;0.372556928229261730134425079086213372647762298583984375;-0.52937373624400063665262905487907119095325469970703125;0.7273236861106806561139137556892819702625274658203125;-0.1655206324634790338024004086037166416645050048828125]
      mask Display: e = 0.06;c1 = [120 150 230]/255;c2 = ([120 150 230]+0)/383;c3 = ([120 150 230]+128)/383;patch([0 1 1 0],[0 0 1 1],c1);patch([0 1 1 1-e 1-e 0+e],[0 0 1 1-e 0+e 0+e],c2);patch([0 0 1 1-e 0+e 0+e],[0 1 1 1-e 1-e 0+e],c3);plot([0 1 1 0 0],[0 0 1 1 0]);disp('weights');
  Mux : Mux  Inputs=15
      mask Display: e = 0.06;c1 = [120 150 230]/255;c2 = ([120 150 230]+0)/383;c3 = ([120 150 230]+128)/383;patch([0 1 1 0],[0 0 1 1],c1);patch([0 1 1 1-e 1-e 0+e],[0 0 1 1-e 0+e 0+e],c2);patch([0 0 1 1-e 0+e 0+e],[0 1 1 1-e 1-e 0+e],c3);plot([0 1 1 0 0],[0 0 1 1 0]);disp('Mux');
  dotprod{1..15} (15 alike) : neural/Weight Functions/dotprod
  "lz{3,2}" : Outport
      mask Display: e = 0.06;c1 = [120 230 180]/255;c2 = ([120 230 180]+0)/(256+128);c3 = ([120 230 180]+128)/(256+128);patch([0 1 1 0],[0 0 1 1],c1);patch([0 1 1 1-e 1-e 0+e],[0 0 1 1-e 0+e 0+e],c2);patch([0 0 1 1-e 0+e 0+e],[0 1 1 1-e 1-e 0+e],c3);plot([0 1 1 0 0],[0 0 1 1 0]);
  wires:
  "IW{3,2}(1,:)'"/1 -> dotprod1/1
  "ad{3,2}"/1 -> dotprod1/2, dotprod2/2, dotprod3/2, dotprod4/2, dotprod5/2, dotprod6/2, dotprod7/2, dotprod8/2, dotprod9/2, dotprod10/2, dotprod11/2, dotprod12/2, dotprod13/2, dotprod14/2, dotprod15/2
  dotprod1/1 -> Mux/1
  "IW{3,2}(2,:)'"/1 -> dotprod2/1
  dotprod2/1 -> Mux/2
  "IW{3,2}(3,:)'"/1 -> dotprod3/1
  dotprod3/1 -> Mux/3
  "IW{3,2}(4,:)'"/1 -> dotprod4/1
  dotprod4/1 -> Mux/4
  "IW{3,2}(5,:)'"/1 -> dotprod5/1
  dotprod5/1 -> Mux/5
  "IW{3,2}(6,:)'"/1 -> dotprod6/1
  dotprod6/1 -> Mux/6
  "IW{3,2}(7,:)'"/1 -> dotprod7/1
  dotprod7/1 -> Mux/7
  "IW{3,2}(8,:)'"/1 -> dotprod8/1
  dotprod8/1 -> Mux/8
  "IW{3,2}(9,:)'"/1 -> dotprod9/1
  dotprod9/1 -> Mux/9
  "IW{3,2}(10,:)'"/1 -> dotprod10/1
  dotprod10/1 -> Mux/10
  "IW{3,2}(11,:)'"/1 -> dotprod11/1
  dotprod11/1 -> Mux/11
  "IW{3,2}(12,:)'"/1 -> dotprod12/1
  dotprod12/1 -> Mux/12
  "IW{3,2}(13,:)'"/1 -> dotprod13/1
  dotprod13/1 -> Mux/13
  "IW{3,2}(14,:)'"/1 -> dotprod14/1
  dotprod14/1 -> Mux/14
  "IW{3,2}(15,:)'"/1 -> dotprod15/1
  dotprod15/1 -> Mux/15
  Mux/1 -> "lz{3,2}"/1

== system nn_fuel_control_4_15/Air Fuel Control Model 1/Feed-Forward Neural Network/Layer 4/Delays 1 ==
  "p{4}" : Inport  PortDimensions=15
      mask Display: e = 0.06;c1 = [120 230 180]/255;c2 = ([120 230 180]+0)/(256+128);c3 = ([120 230 180]+128)/(256+128);patch([0 1 1 0],[0 0 1 1],c1);patch([0 1 1 1-e 1-e 0+e],[0 0 1 1-e 0+e 0+e],c2);patch([0 0 1 1-e 0+e 0+e],[0 1 1 1-e 1-e 0+e],c3);plot([0 1 1 0 0],[0 0 1 1 0]);
  mux : Mux  Inputs=1
      mask Display: e = 0.06;c1 = [120 150 230]/255;c2 = ([120 150 230]+0)/383;c3 = ([120 150 230]+128)/383;patch([0 1 1 0],[0 0 1 1],c1);patch([0 1 1 1-e 1-e 0+e],[0 0 1 1-e 0+e 0+e],c2);patch([0 0 1 1-e 0+e 0+e],[0 1 1 1-e 1-e 0+e],c3);plot([0 1 1 0 0],[0 0 1 1 0]);disp('Mux')
  "pd{4,3}" : Outport
      mask Display: e = 0.06;c1 = [120 230 180]/255;c2 = ([120 230 180]+0)/(256+128);c3 = ([120 230 180]+128)/(256+128);patch([0 1 1 0],[0 0 1 1],c1);patch([0 1 1 1-e 1-e 0+e],[0 0 1 1-e 0+e 0+e],c2);patch([0 0 1 1-e 0+e 0+e],[0 1 1 1-e 1-e 0+e],c3);plot([0 1 1 0 0],[0 0 1 1 0]);
  wires:
  "p{4}"/1 -> mux/1
  mux/1 -> "pd{4,3}"/1
